simulink model "HIGH_LEVEL_MODULATOR"  (R2021b)
settings: Solver=VariableStepAuto  StartTime=0.0  StopTime=1  RelTol=1e-3
libraries: commdigbbndpm3 x2, commchan3 x1, commsink2 x1, dspsrcs4 x1, commrandsrc3 x1
settings Model: Creator=caccolillo  LastModifiedBy=caccolillo

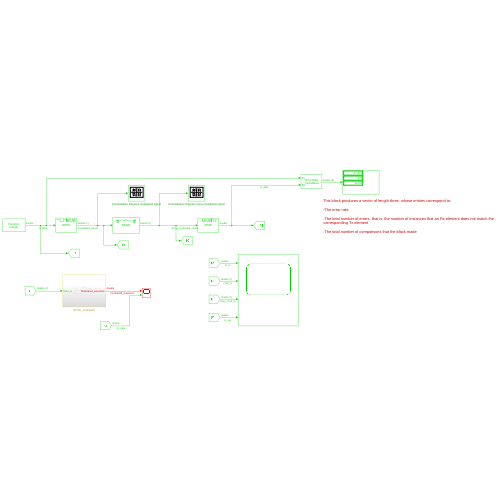
[thumbnail: Simulink's stored preview of the top-level diagram]
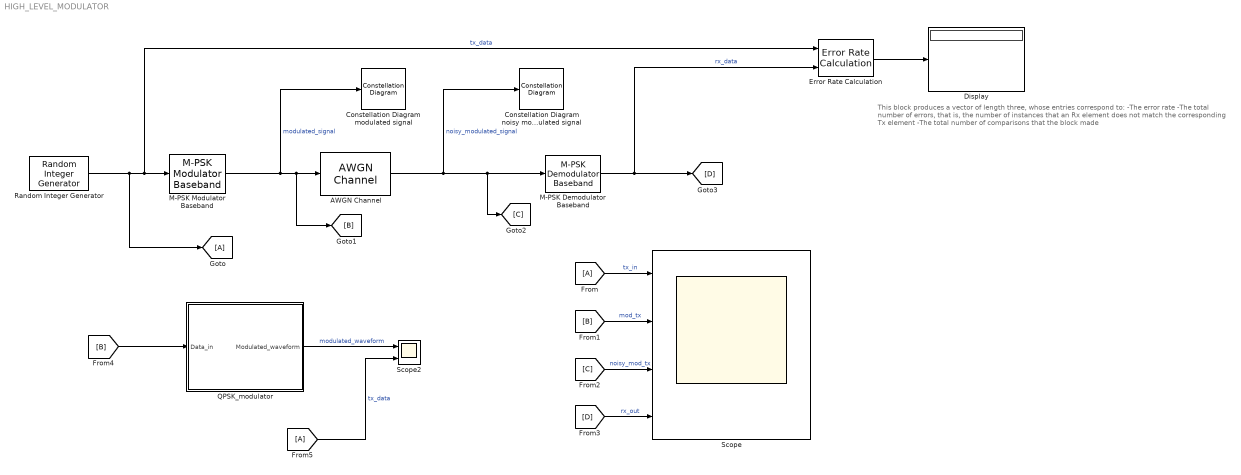
== system HIGH_LEVEL_MODULATOR ==
  note: This block produces a vector of length three, whose entries correspond to:
      |
      | -The error rate
      |
      | -The total number of errors, that is, the number of instances that an Rx element does not match the corresponding Tx element
      |
      | -The total number of comparisons that the block made
  AWGN Channel : commchan3/AWGN Channel  InputProcessing=Columns as channels (frame based)  seed=67  noiseMode="Signal to noise ratio  (Eb/No)"  EbNodB=10  EsNodB=-100  SNRdB=10  bitsPerSym=1  Ps=1  Tsym=1  variance=1
  Constellation Diagram modulated signal : ConstellationDiagram
  Constellation Diagram noisy modulated signal : ConstellationDiagram
  Display : Display
  Error Rate Calculation : commsink2/Error Rate Calculation  N=0  st_delay=0  cp_mode=Entire frame  subframe=[]  PMode=Port  WsName=ErrorVec  RsMode2=off  stop=off  numErr=100  maxBits=1e6
  M-PSK Demodulator Baseband : commdigbbndpm3/M-PSK Demodulator Baseband  M=4  OutType=Integer  DecType=Hard decision  VarSource=Dialog  Variance=1  Dec=Gray  Mapping=[0:7]  Ph=pi/4  outDtype1=Inherit via internal rule  outDtype2=Inherit via internal rule  derotateFactorWordLen=16  derotateFactorDataTypeStr=Inherit: Same word length as input  derotateFactorLastDataTypeStr=Inherit: Same word length as input
  M-PSK Modulator Baseband : commdigbbndpm3/M-PSK Modulator Baseband  M=4  InType=Integer  Enc=Gray  Mapping=[0:7]  Ph=pi/4  outDtype=double  outWordLen=16  outUDDataType=sfix(16)  outFracLenMode=Best precision  outFracLen=15  outDataTypeStr=double  outLastDataTypeStr=double
  QPSK_modulator : Subsystem
  Random Integer Generator : commrandsrc3/Random Integer Generator  SetSize=4  SeedSource=Auto  Seed=0  SampleTime=1/10000  SamplesPerFrame=1  OutputDataType=double  SimulateUsing=Interpreted execution
  Scope : Scope  NumInputPorts=4
  Scope2 : Scope  NumInputPorts=2
  wires:
  M-PSK Modulator Baseband/1 -> Constellation Diagram modulated signal/1, [B], AWGN Channel/1  "modulated_signal"
  Random Integer Generator/1 -> [A], Error Rate Calculation/1, M-PSK Modulator Baseband/1  "tx_data"
  M-PSK Demodulator Baseband/1 -> [D], Error Rate Calculation/2  "rx_data"
  AWGN Channel/1 -> Constellation Diagram noisy modulated signal/1, [C], M-PSK Demodulator Baseband/1  "noisy_modulated_signal"
  Error Rate Calculation/1 -> Display/1
  [A] -> Scope/1  "tx_in"
  [B] -> Scope/2  "mod_tx"
  [C] -> Scope/3  "noisy_mod_tx"
  [D] -> Scope/4  "rx_out"
  [B] -> QPSK_modulator/1(Data_in)
  QPSK_modulator/1(Modulated_waveform) -> Scope2/1  "modulated_waveform"
  [A] -> Scope2/2  "tx_data"

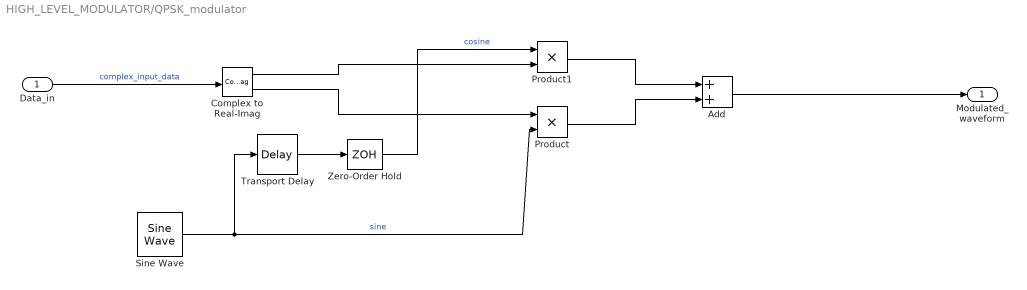
== system HIGH_LEVEL_MODULATOR/QPSK_modulator ==
  Data_in : Inport
  Add : Sum
  Complex to Real-Imag : ComplexToRealImag
  Product : Product
  Product1 : Product
  Sine Wave : dspsrcs4/Sine Wave  Amplitude=1  Frequency=20000  Phase=0  SampleMode=Discrete  OutComplex=Real  CompMethod=Table lookup  TableSize=Speed  SampleTime=1/200000  SamplesPerFrame=1  ResetState=Restart at time zero  OutputFrames=off  dataType=double  wordLen=16  udDataType=sfix(16)  fracBitsMode=Best precision  numFracBits=15  OutDataTypeStr=double  LastOutDataTypeStr=double
  Transport Delay : TransportDelay  DelayTime=1 / (4 * 20000)
  Zero-Order Hold : ZeroOrderHold  SampleTime=1/200000
  Modulated_waveform : Outport
  wires:
  Complex to Real-Imag/1 -> Product1/2
  Product/1 -> Add/2
  Transport Delay/1 -> Zero-Order Hold/1
  Sine Wave/1 -> Transport Delay/1, Product/2  "sine"
  Add/1 -> Modulated_waveform/1
  Zero-Order Hold/1 -> Product1/1  "cosine"
  Product1/1 -> Add/1
  Data_in/1 -> Complex to Real-Imag/1  "complex_input_data"
  Complex to Real-Imag/2 -> Product/1
